simulink model "Problem_1_Part_C3"  (R2018b)
settings: Solver=FixedStepAuto  StartTime=0.0  StopTime=600  FixedStep=0.002  RelTol=1e-3
InitFcn:
  | Initial_Data
values from neighbouring files (symbols this model uses):
  au = normrnd(mu2,sigma2)    [Velocity_Acceleration_Measurement_Uncertinty.m]
  Vu = normrnd(mu1,sigma1)    [Velocity_Acceleration_Measurement_Uncertinty.m]
undefined symbols (not defined in the file or in its folder): errorV, Gamma0, GM, Long0, R0, Rf, V0
libraries: vrlib x2, simulink x1, simulink_extras x1
settings Model: Creator=User  LastModifiedBy=User
settings SolverCC: AlgebraicLoopSolver=LineSearch

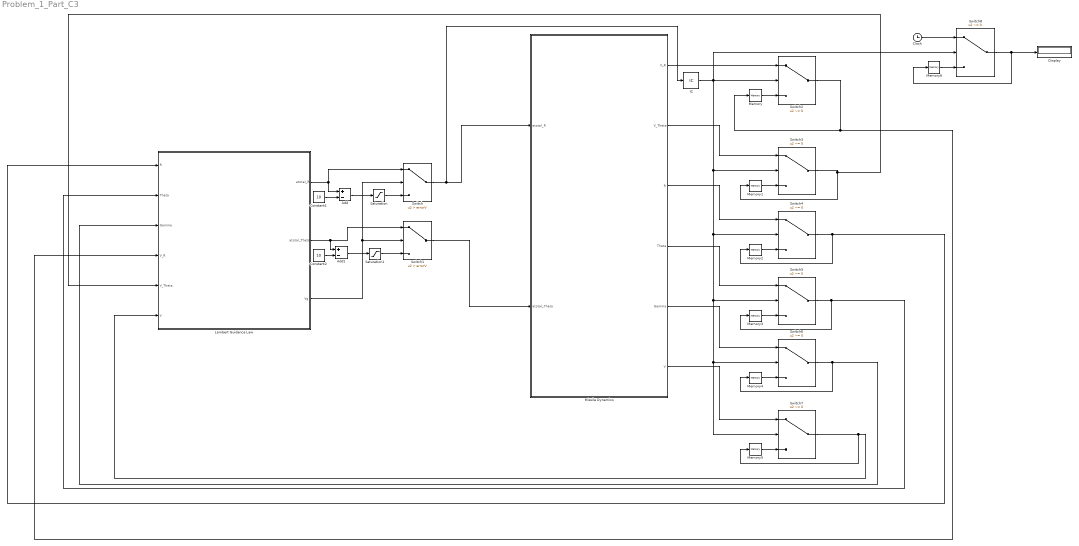
== system Problem_1_Part_C3 ==
  Add : Sum  Inputs=+-
  Add1 : Sum  Inputs=+-
  Clock : Clock
  Constant1 : Constant  Value=10
  Constant2 : Constant  Value=10
  Display : Display
  IC : InitialCondition  Value=0.01
  Lambert Guidance Law : Subsystem
  Memory{,1..6} (7 alike) : Memory
  Missile Dynamics : Subsystem
  Saturation : Saturate  UpperLimit=inf  LowerLimit=0
  Saturation1 : Saturate  UpperLimit=inf  LowerLimit=0
  Switch : Switch  Criteria=u2 > Threshold  Threshold=errorV
  Switch1 : Switch  Criteria=u2 > Threshold  Threshold=errorV
  Switch{2..8} (7 alike) : Switch  Criteria=u2 ~= 0  Threshold=45.054
  wires:
  Lambert Guidance Law/3(Vg) -> Switch1/2, Switch/2
  Lambert Guidance Law/1(atotal_R) -> Add/1, Switch/1
  Switch1/1 -> Missile Dynamics/2(atotal_Theta)
  Memory5/1 -> Switch7/3
  Switch2/1 -> Memory/1, Lambert Guidance Law/4(V_R)
  Memory3/1 -> Switch5/3
  Memory2/1 -> Switch4/3
  IC/1 -> Switch8/2, Switch4/2, Switch7/2, Switch6/2, Switch5/2, Switch3/2, Switch2/2
  Memory4/1 -> Switch6/3
  Memory1/1 -> Switch3/3
  Missile Dynamics/4(Theta) -> Switch5/1
  Missile Dynamics/1(V_R) -> Switch2/1
  Missile Dynamics/5(Gamma) -> Switch6/1
  Memory/1 -> Switch2/3
  Switch4/1 -> Memory2/1, Lambert Guidance Law/1(R)
  Missile Dynamics/6(V) -> Switch7/1
  Switch5/1 -> Memory3/1, Lambert Guidance Law/2(Theta)
  Missile Dynamics/3(R) -> Switch4/1
  Switch/1 -> IC/1, Missile Dynamics/1(atotal_R)
  Switch3/1 -> Memory1/1, Lambert Guidance Law/5(V_Theta)
  Switch7/1 -> Memory5/1, Lambert Guidance Law/6(V)
  Missile Dynamics/2(V_Theta) -> Switch3/1
  Switch6/1 -> Memory4/1, Lambert Guidance Law/3(Gamma)
  Constant1/1 -> Add/2
  Add/1 -> Saturation/1
  Saturation/1 -> Switch/3
  Lambert Guidance Law/2(atotal_Theta) -> Add1/1, Switch1/1
  Saturation1/1 -> Switch1/3
  Add1/1 -> Saturation1/1
  Constant2/1 -> Add1/2
  Switch8/1 -> Display/1, Memory6/1
  Clock/1 -> Switch8/1
  Memory6/1 -> Switch8/3

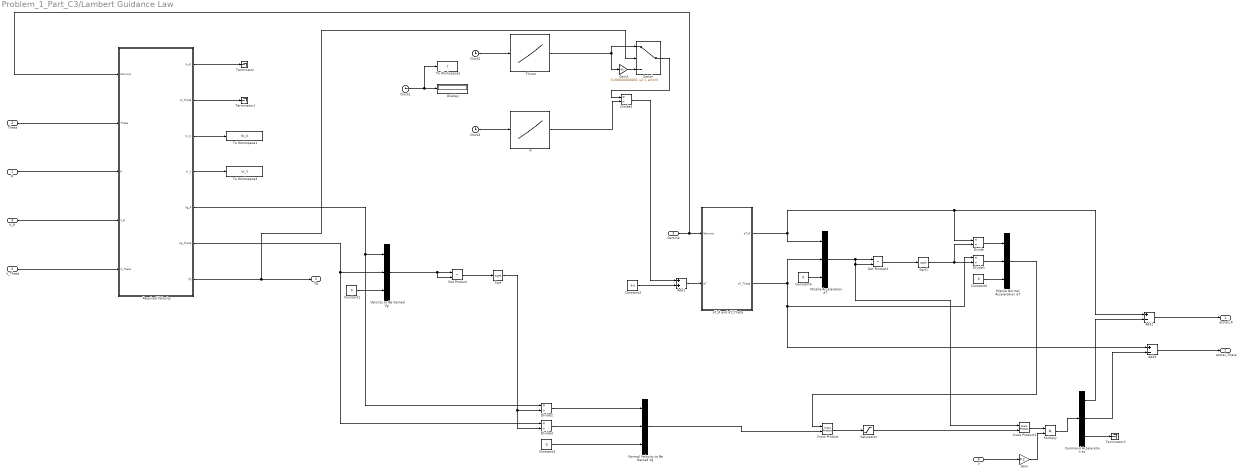
== system Problem_1_Part_C3/Lambert Guidance Law ==
  R : Inport
  Theta : Inport  Port=2
  Gamma : Inport  Port=3
  V_R : Inport  Port=4
  V_Theta : Inport  Port=5
  V : Inport  Port=6
  Add1 : Sum
  Add2 : Sum  Inputs=+-
  Add3 : Sum  Inputs=+-
  Clock1 : Clock
  Clock2 : Clock
  Clock3 : Clock
  Command Acceleration ac : Demux  Outputs=3
  Constant{1,3..5} (4 alike) : Constant  Value=0
  Constant2 : Constant  Value=au
  Cross Product : vrlib/Utilities/Cross Product
      settings: SourceProductBaseCode=VR
  Cross Product1 : vrlib/Utilities/Cross Product
      settings: SourceProductBaseCode=VR
  Display : Display
  Divide{,1..4} (5 alike) : Product  Inputs=*/
  Dot Product : DotProduct  InputSameDT=on  OutDataTypeStr=Inherit: Inherit via internal rule
  Dot Product1 : DotProduct  InputSameDT=on  OutDataTypeStr=Inherit: Inherit via internal rule
  Gain : Gain  Gain=0.2
  Gain1 : Gain  Gain=0.000000000001
  Missile Acceleration aT : Mux  Inputs=3
  Missile Normal Acceleration aT : Mux  Inputs=3
  Multiply : Product
  Normal Velocity to Be Gained Vg : Mux  Inputs=3
  Required Velocity : MATLAB Function  TreatAsAtomicUnit=on
  Saturation : Saturate  UpperLimit=1*pi/180  LowerLimit=-1*pi/180
  Sqrt : Sqrt  SaturateOnIntegerOverflow=on
  Sqrt1 : Sqrt  SaturateOnIntegerOverflow=on
  Switch : Switch  Criteria=u2 > Threshold  Threshold=errorV
  Terminator : Terminator
  Terminator1 : Terminator
  Terminator2 : Terminator
  Thrust : Lookup_n-D  NumberOfTableDimensions=1  BreakpointsForDimension1=[0;60;61]  Table=[160000;160000;160000]  InternalRulePriority=Speed  RndMeth=Simplest  InputSameDT=on
  To Workspace1 : ToWorkspace  VariableName=Vr_X  SampleTime=-1
  To Workspace2 : ToWorkspace  VariableName=t  SampleTime=-1
  To Workspace3 : ToWorkspace  VariableName=Vr_Y  SampleTime=-1
  Velocity to Be Gained Vg : Mux  Inputs=3
  aT_R and aT_Theta : MATLAB Function  TreatAsAtomicUnit=on
  m : Lookup_n-D  NumberOfTableDimensions=1  BreakpointsForDimension1=[0;60;61]  Table=[3000;320;320]  InternalRulePriority=Speed  RndMeth=Simplest  InputSameDT=on
  atotal_R : Outport
  atotal_Theta : Outport  Port=2
  Vg : Outport  Port=3
  wires:
  Theta/1 -> Required Velocity/2(Theta)
  R/1 -> Required Velocity/3(R)
  Velocity to Be Gained Vg/1 -> Dot Product/2, Dot Product/1
  Dot Product/1 -> Sqrt/1
  aT_R and aT_Theta/1(aT_R) -> Add2/1, Divide/1, Missile Acceleration aT/1
  aT_R and aT_Theta/2(aT_Theta) -> Divide1/1, Add3/1, Missile Acceleration aT/2
  Missile Acceleration aT/1 -> Cross Product1/1, Dot Product1/2, Dot Product1/1
  Dot Product1/1 -> Sqrt1/1
  Sqrt1/1 -> Divide1/2, Divide/2
  Divide/1 -> Missile Normal Acceleration aT/1
  Divide1/1 -> Missile Normal Acceleration aT/2
  Divide3/1 -> Normal Velocity to Be Gained Vg/2
  Sqrt/1 -> Divide3/2, Divide2/2
  Divide2/1 -> Normal Velocity to Be Gained Vg/1
  Required Velocity/6(Vg_Theta) -> Divide3/1, Velocity to Be Gained Vg/2
  Normal Velocity to Be Gained Vg/1 -> Cross Product/2
  Missile Normal Acceleration aT/1 -> Cross Product/1
  Add2/1 -> atotal_R/1
  Add3/1 -> atotal_Theta/1
  Command Acceleration ac/1 -> Add2/2
  Command Acceleration ac/2 -> Add3/2
  Constant1/1 -> Velocity to Be Gained Vg/3
  Constant3/1 -> Normal Velocity to Be Gained Vg/3
  Constant4/1 -> Missile Acceleration aT/3
  Constant5/1 -> Missile Normal Acceleration aT/3
  Command Acceleration ac/3 -> Terminator2/1
  Cross Product/1 -> Saturation/1
  Gain/1 -> Multiply/2
  Multiply/1 -> Command Acceleration ac/1
  V_Theta/1 -> Required Velocity/5(V_Theta)
  Required Velocity/2(Vr_Theta) -> Terminator1/1
  Required Velocity/1(Vr_R) -> Terminator/1
  Required Velocity/3(Vr_X) -> To Workspace1/1
  Required Velocity/4(Vr_Y) -> To Workspace3/1
  Required Velocity/5(Vg_R) -> Divide2/1, Velocity to Be Gained Vg/1
  m/1 -> Divide4/2
  Clock3/1 -> m/1
  Clock2/1 -> Thrust/1
  Thrust/1 -> Gain1/1, Switch/1
  Clock1/1 -> To Workspace2/1, Display/1
  Saturation/1 -> Cross Product1/2
  Cross Product1/1 -> Multiply/1
  Required Velocity/7(Vg) -> Vg/1, Switch/2
  Gamma/1 -> Required Velocity/1(Gamma), aT_R and aT_Theta/1(Gamma)
  V_R/1 -> Required Velocity/4(V_R)
  V/1 -> Gain/1
  Switch/1 -> Divide4/1
  Gain1/1 -> Switch/3
  Constant2/1 -> Add1/2
  Add1/1 -> aT_R and aT_Theta/2(aT)
  Divide4/1 -> Add1/1

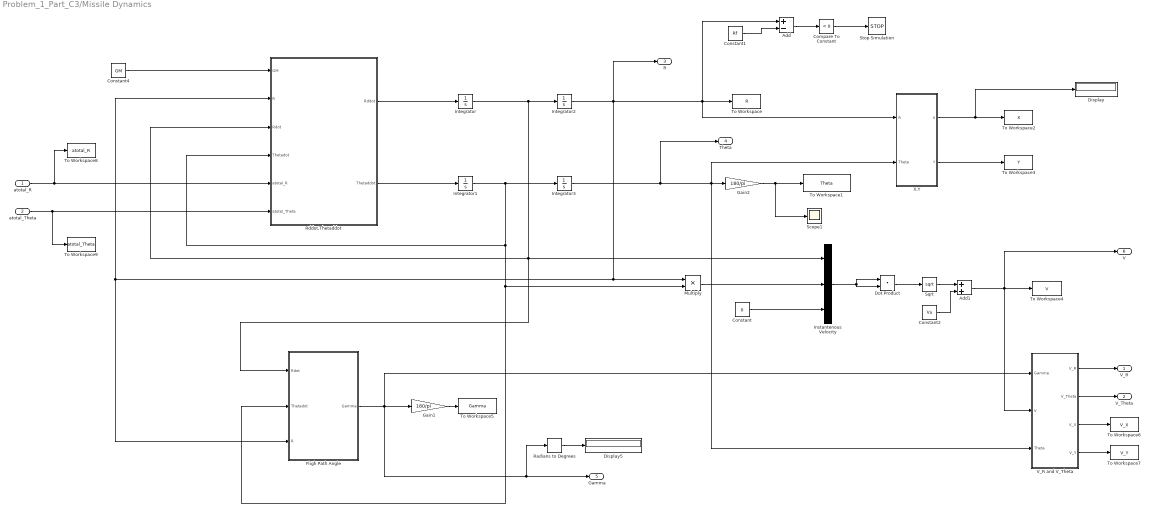
== system Problem_1_Part_C3/Missile Dynamics ==
  atotal_R : Inport
  atotal_Theta : Inport  Port=2
  Add : Sum  Inputs=+-
  Add1 : Sum
  Compare To Constant : simulink/Logic and Bit Operations/Compare To Constant  relop=<  const=0  OutDataTypeStr=boolean
  Constant : Constant  Value=0
  Constant1 : Constant  Value=Rf
  Constant2 : Constant  Value=Vu
  Constant4 : Constant  Value=GM
  Display : Display
  Display5 : Display
  Dot Product : DotProduct  InputSameDT=on  OutDataTypeStr=Inherit: Inherit via internal rule
  Fligh Path Angle : MATLAB Function  TreatAsAtomicUnit=on
  Gain1 : Gain  Gain=180/pi
  Gain2 : Gain  Gain=180/pi
  Instantenous Velocity : Mux  Inputs=3
  Integrator : Integrator  InitialCondition=V0*sin(Gamma0)
  Integrator1 : Integrator  InitialCondition=(V0*cos(Gamma0))/R0
  Integrator2 : Integrator  InitialCondition=R0
  Integrator3 : Integrator  InitialCondition=Long0*pi/180
  Multiply : Product
  Radians to Degrees : simulink_extras/Transformations/Radians to Degrees
  Rddot,Thetaddot : MATLAB Function  TreatAsAtomicUnit=on
  Scope1 : Scope
  Sqrt : Sqrt  SaturateOnIntegerOverflow=on
  Stop Simulation : Stop
  To Workspace : ToWorkspace  VariableName=R  SampleTime=-1
  To Workspace1 : ToWorkspace  VariableName=Theta  SampleTime=-1
  To Workspace2 : ToWorkspace  VariableName=X  SampleTime=-1
  To Workspace3 : ToWorkspace  VariableName=Y  SampleTime=-1
  To Workspace4 : ToWorkspace  VariableName=V  SampleTime=-1
  To Workspace5 : ToWorkspace  VariableName=Gamma  SampleTime=-1
  To Workspace6 : ToWorkspace  VariableName=V_X  SampleTime=-1
  To Workspace7 : ToWorkspace  VariableName=V_Y  SampleTime=-1
  To Workspace8 : ToWorkspace  VariableName=atotal_R  SampleTime=-1
  To Workspace9 : ToWorkspace  VariableName=atotal_Theta  SampleTime=-1
  V_R and V_Theta : MATLAB Function  TreatAsAtomicUnit=on
  X,Y : MATLAB Function  TreatAsAtomicUnit=on
  V_R : Outport
  V_Theta : Outport  Port=2
  R : Outport  Port=3
  Theta : Outport  Port=4
  Gamma : Outport  Port=5
  V : Outport  Port=6
  wires:
  Rddot,Thetaddot/2(Thetaddot) -> Integrator1/1
  Rddot,Thetaddot/1(Rddot) -> Integrator/1
  Integrator/1 -> Fligh Path Angle/1(Rdot), Rddot,Thetaddot/3(Rdot), Instantenous Velocity/1, Integrator2/1
  Integrator1/1 -> Integrator3/1, Fligh Path Angle/2(Thetadot), Multiply/2, Rddot,Thetaddot/4(Thetadot)
  Integrator3/1 -> Theta/1, Gain2/1, V_R and V_Theta/3(Theta), X,Y/2(Theta)
  Integrator2/1 -> Add/1, To Workspace/1, X,Y/1(R), R/1, Multiply/1, Rddot,Thetaddot/2(R), Fligh Path Angle/3(R)
  X,Y/1(X) -> Display/1, To Workspace2/1
  X,Y/2(Y) -> To Workspace3/1
  Constant4/1 -> Rddot,Thetaddot/1(GM)
  Fligh Path Angle/1(Gamma) -> Gain1/1, Radians to Degrees/1, Gamma/1, V_R and V_Theta/1(Gamma)
  Dot Product/1 -> Sqrt/1
  Instantenous Velocity/1 -> Dot Product/1, Dot Product/2
  Gain1/1 -> To Workspace5/1
  Multiply/1 -> Instantenous Velocity/2
  Gain2/1 -> Scope1/1, To Workspace1/1
  V_R and V_Theta/1(V_R) -> V_R/1
  V_R and V_Theta/2(V_Theta) -> V_Theta/1
  atotal_R/1 -> To Workspace8/1, Rddot,Thetaddot/5(atotal_R)
  atotal_Theta/1 -> To Workspace9/1, Rddot,Thetaddot/6(atotal_Theta)
  Constant/1 -> Instantenous Velocity/3
  V_R and V_Theta/3(V_X) -> To Workspace6/1
  V_R and V_Theta/4(V_Y) -> To Workspace7/1
  Radians to Degrees/1 -> Display5/1
  Add/1 -> Compare To Constant/1
  Constant1/1 -> Add/2
  Compare To Constant/1 -> Stop Simulation/1
  Constant2/1 -> Add1/2
  Sqrt/1 -> Add1/1
  Add1/1 -> To Workspace4/1, V/1, V_R and V_Theta/2(V)

== matlab function Problem_1_Part_C3/Missile Dynamics/Fligh Path Angle ==
  data: Rdot input; Gamma output; Thetadot input; R input
function Gamma = fcn(Rdot,Thetadot,R)

Gamma = atan((Rdot)/(R*Thetadot));

== matlab function Problem_1_Part_C3/Missile Dynamics/X,Y ==
  data: R input; X output; Theta input; Y output
function [X,Y] = fcn(R,Theta)

X = R*cos(Theta);
Y = R*sin(Theta);

== matlab function Problem_1_Part_C3/Missile Dynamics/Rddot,Thetaddot ==
  data: GM input; Rddot output; R input; Rdot input; Thetadot input; Thetaddot output; atotal_R input; atotal_Theta input
function [Rddot,Thetaddot]  = fcn(GM,R,Rdot,Thetadot,atotal_R,atotal_Theta)

Rddot = R*Thetadot^2 - (GM)/(R^2) + atotal_R;
Thetaddot = (-2*Rdot*Thetadot + atotal_Theta)/(R);

== matlab function Problem_1_Part_C3/Missile Dynamics/V_R and V_Theta ==
  data: Gamma input; V_R output; V input; V_Theta output; Theta input; V_X output; V_Y output
function [V_R,V_Theta,V_X,V_Y] = fcn(Gamma,V,Theta)

V_R = V*sin(Gamma);
V_X = V*sin(Gamma)*cos(Theta);
V_Y = V*sin(Gamma)*sin(Theta);
V_Theta = V*cos(Gamma);

== matlab function Problem_1_Part_C3/Lambert Guidance Law/aT_R and aT_Theta ==
  data: Gamma input; aT_R output; aT input; aT_Theta output
function [aT_R,aT_Theta] = fcn(Gamma,aT)

aT_R = aT*sin(Gamma);
aT_Theta = aT*cos(Gamma);

== matlab function Problem_1_Part_C3/Lambert Guidance Law/Required Velocity ==
  data: Gamma input; Theta input; R input; V_R input; V_Theta input; Vr_R output; Vr_Theta output; Vr_X output; Vr_Y output; Vg_R output; Vg_Theta output; Vg output
function [Vr_R,Vr_Theta,Vr_X,Vr_Y,Vg_R,Vg_Theta,Vg] = fcn(Gamma,Theta,R,V_R,V_Theta)

%% Lambert
Longf = 50*pi/180; %degree%
Rf = 6371000; %m%
GM = 3.986004418*(10^14); %m^3/s^2%
Phi = (Longf - Theta);%rad%  
Vr = sqrt( (GM*( 1-cos(Phi)))/((R*cos(Gamma))*((R*cos(Gamma))/(Rf) - cos(Phi+Gamma))) );

Vr_R = Vr*sin(Gamma);
Vr_Theta = Vr*cos(Gamma);
Vr_X = Vr*sin(Gamma)*cos(Theta);
Vr_Y = Vr*sin(Gamma)*sin(Theta);
Vg_R = Vr_R - V_R;
Vg_Theta = Vr_Theta - V_Theta;
Vg = sqrt( (Vg_R)^2 + (Vg_Theta)^2 );
